simulink model "Equation_of_motion_sim"  (R2022b)
settings: Solver=FixedStepAuto  StartTime=0.0  StopTime=time_sim(end)  FixedStep=1/100  RelTol=1e-3
undefined symbols (not defined in the file or in its folder): DiscIntNeverNeededParam, init_euler
libraries: sharedtransform x1
settings Model: Creator=ohad1  LastModifiedBy=ohad1

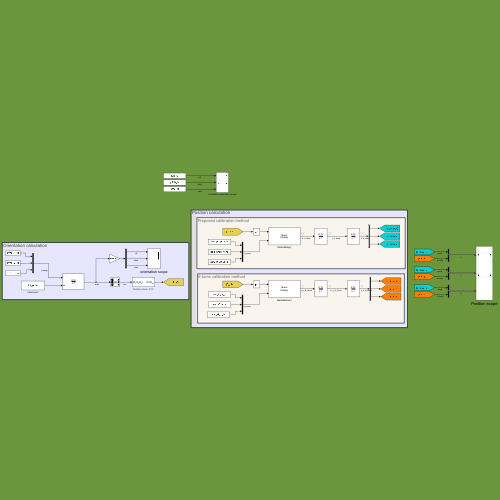
[thumbnail: Simulink's stored preview of the top-level diagram]
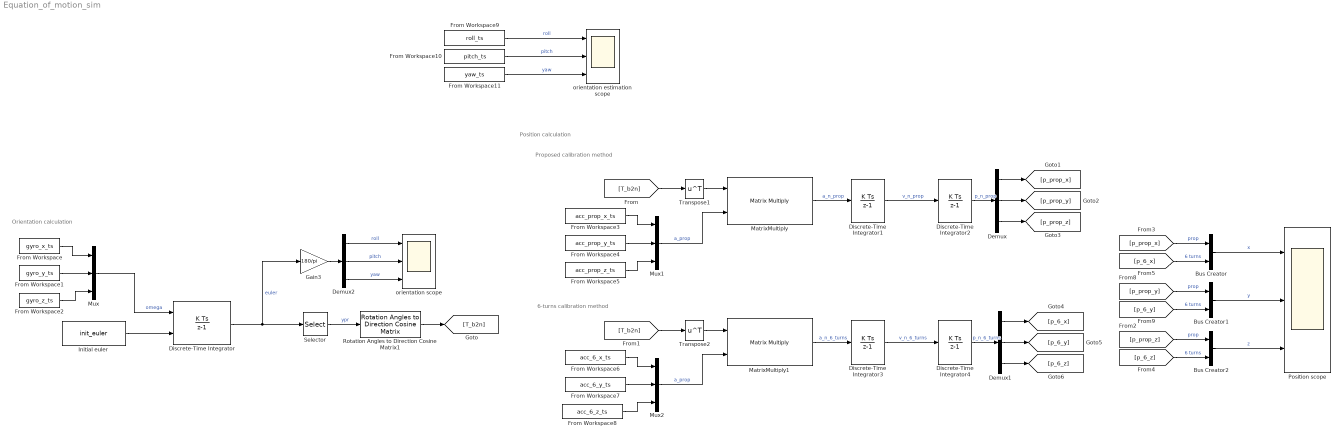
== system Equation_of_motion_sim ==
  note: 6-turns calibration method
  note: Proposed calibration method
  note: Position calculation
  note: Orientation calculation
  Bus Creator : BusCreator  Inputs=2
  Bus Creator1 : BusCreator  Inputs=2
  Bus Creator2 : BusCreator  Inputs=2
  Demux : Demux  Outputs=3
  Demux1 : Demux  Outputs=3
  Demux2 : Demux  Outputs=3
  Discrete-Time Integrator : DiscreteIntegrator  InitialConditionSource=external  SampleTime=-1  ICPrevOutput=DiscIntNeverNeededParam  ICPrevScaledInput=DiscIntNeverNeededParam
  Discrete-Time Integrator{1..4} (4 alike) : DiscreteIntegrator  SampleTime=-1  ICPrevOutput=DiscIntNeverNeededParam  ICPrevScaledInput=DiscIntNeverNeededParam
  From Workspace : FromWorkspace  VariableName=gyro_x_ts
  From Workspace1 : FromWorkspace  VariableName=gyro_y_ts
  From Workspace10 : FromWorkspace  VariableName=pitch_ts
  From Workspace11 : FromWorkspace  VariableName=yaw_ts
  From Workspace2 : FromWorkspace  VariableName=gyro_z_ts
  From Workspace3 : FromWorkspace  VariableName=acc_prop_x_ts
  From Workspace4 : FromWorkspace  VariableName=acc_prop_y_ts
  From Workspace5 : FromWorkspace  VariableName=acc_prop_z_ts
  From Workspace6 : FromWorkspace  VariableName=acc_6_x_ts
  From Workspace7 : FromWorkspace  VariableName=acc_6_y_ts
  From Workspace8 : FromWorkspace  VariableName=acc_6_z_ts
  From Workspace9 : FromWorkspace  VariableName=roll_ts
  Gain3 : Gain  Gain=180/pi
  Initial euler : Constant  Value=init_euler
  MatrixMultiply : Product  Multiplication=Matrix(*)
  MatrixMultiply1 : Product  Multiplication=Matrix(*)
  Mux : Mux  Inputs=3
  Mux1 : Mux  Inputs=3
  Mux2 : Mux  Inputs=3
  Position scope : Scope  NumInputPorts=3
  Rotation Angles to Direction Cosine Matrix1 : sharedtransform/Rotation Angles to Direction Cosine Matrix  rotationOrder=ZYX  aMode=aMode
  Selector : Selector  InputPortWidth=3  IndexOptions=Index vector (dialog)  Indices=[3 2 1]  OutputSizes=1
  Transpose1 : Math  Operator=transpose
  Transpose2 : Math  Operator=transpose
  orientation estimation scope : Scope  NumInputPorts=3
  orientation scope : Scope  NumInputPorts=3
  wires:
  Initial euler/1 -> Discrete-Time Integrator/2
  From Workspace/1 -> Mux/1
  From Workspace1/1 -> Mux/2
  From Workspace2/1 -> Mux/3
  Mux/1 -> Discrete-Time Integrator/1  "omega"
  Selector/1 -> Rotation Angles to Direction Cosine Matrix1/1  "ypr"
  Rotation Angles to Direction Cosine Matrix1/1 -> [T_b2n]
  [T_b2n] -> Transpose1/1
  Transpose1/1 -> MatrixMultiply/1
  Mux1/1 -> MatrixMultiply/2  "a_prop"
  From Workspace3/1 -> Mux1/1
  From Workspace4/1 -> Mux1/2
  From Workspace5/1 -> Mux1/3
  MatrixMultiply/1 -> Discrete-Time Integrator1/1  "a_n_prop"
  Discrete-Time Integrator1/1 -> Discrete-Time Integrator2/1  "v_n_prop"
  Discrete-Time Integrator2/1 -> Demux/1  "p_n_prop"
  Discrete-Time Integrator4/1 -> Demux1/1  "p_n_6_turns"
  Discrete-Time Integrator3/1 -> Discrete-Time Integrator4/1  "v_n_6_turns"
  MatrixMultiply1/1 -> Discrete-Time Integrator3/1  "a_n_6_turns"
  From Workspace8/1 -> Mux2/3
  From Workspace7/1 -> Mux2/2
  From Workspace6/1 -> Mux2/1
  Mux2/1 -> MatrixMultiply1/2  "a_prop"
  Transpose2/1 -> MatrixMultiply1/1
  [T_b2n] -> Transpose2/1
  Demux/1 -> [p_prop_x]
  Demux/2 -> [p_prop_y]
  Demux/3 -> [p_prop_z]
  Demux1/3 -> [p_6_z]
  Demux1/2 -> [p_6_y]
  Demux1/1 -> [p_6_x]
  Bus Creator/1 -> Position scope/1  "x"
  [p_prop_x] -> Bus Creator/1  "prop"
  [p_6_x] -> Bus Creator/2  "6 turns"
  [p_6_y] -> Bus Creator1/2  "6 turns"
  [p_prop_y] -> Bus Creator1/1  "prop"
  Bus Creator1/1 -> Position scope/2  "y"
  Bus Creator2/1 -> Position scope/3  "z"
  [p_prop_z] -> Bus Creator2/1  "prop"
  [p_6_z] -> Bus Creator2/2  "6 turns"
  Demux2/1 -> orientation scope/1  "roll"
  Demux2/2 -> orientation scope/2  "pitch"
  Demux2/3 -> orientation scope/3  "yaw"
  Gain3/1 -> Demux2/1
  From Workspace11/1 -> orientation estimation scope/3  "yaw"
  From Workspace10/1 -> orientation estimation scope/2  "pitch"
  From Workspace9/1 -> orientation estimation scope/1  "roll"
  Discrete-Time Integrator/1 -> Gain3/1, Selector/1  "euler"
